simulink model "sim_quadrotor"  (R2015a)
settings: Solver=ode3  StartTime=0  StopTime=20  FixedStep=sampleTime_qcsim  MaxStep=0.1  RelTol=1e-3
InitFcn:
  | % load parameters of the default quadrotor
  | disp('Quadrotor parameters loaded by InitFcn')
  | paramsFilters %load mdl_quadcopter as well!
  | 
  | % change to Simulation folder if in data folder
  | cd([matlabpath '/Simulation']);
values from neighbouring files (symbols this model uses):
  altEstim =     [linsys1_pset3.mat]
  controlParams =     [linsys1_pset3.mat]
  ofhandle =     [linsys1_pset3.mat]
  quad =     [linsys1_pset3.mat]
  quadEDT =     [linsys1_pset3.mat]
  sampleTime_qcsim = 0.005    [linsys1_pset3.mat]
  vishandle =     [linsys1_pset3.mat]
undefined symbols (not defined in the file or in its folder): Discrete, K_poleplace, Time
libraries: simulink x26, ctrlSharedLib x3, commnoisgen2 x1
(part 2 of 2)

== system sim_quadrotor/DroneRS_Compensator/Estimator/EstimatorXYPosition/EstimatorXYPosition/OutlierHandling ==
  att_estimin : Inport
  posVIS_datin : Inport  Port=2
  pos_estim : Inport  Port=3
  Add1 : Sum  Inputs=+-
  Demux6 : Demux  Outputs=3
  Logical Operator3 : Logic  Inputs=4  AllPortsSameDT=off  OutDataTypeStr=boolean
  SelectX : Selector  InputPortWidth=4  Indices=[1]
  SelectXY : Selector  InputPortWidth=4  Indices=[1 2]
  abs : MATLAB Function  TreatAsAtomicUnit=on
  checkPosavailable : simulink/Logic and Bit Operations/Compare To Constant  relop=~=  const=-99  OutDataTypeStr=boolean
  maxp3 : simulink/Logic and Bit Operations/Compare To Constant  relop=<=  const=vishandle.att_UpperLimit  OutDataTypeStr=boolean
  maxq3 : simulink/Logic and Bit Operations/Compare To Constant  relop=<=  const=vishandle.att_UpperLimit  OutDataTypeStr=boolean
  planarjumpsVISPOS : simulink/Logic and Bit Operations/Compare To Constant  relop=<  const=vishandle.deltaXY  OutDataTypeStr=boolean
  enable_flag : Outport
  wires:
  att_estimin/1 -> Demux6/1
  posVIS_datin/1 -> SelectXY/1, SelectX/1
  SelectX/1 -> checkPosavailable/1
  checkPosavailable/1 -> Logical Operator3/1
  Logical Operator3/1 -> enable_flag/1
  Demux6/2 -> maxp3/1
  Demux6/3 -> maxq3/1
  maxp3/1 -> Logical Operator3/2
  maxq3/1 -> Logical Operator3/3
  SelectXY/1 -> Add1/1
  Add1/1 -> abs/1(vec)
  pos_estim/1 -> Add1/2
  abs/1(y) -> planarjumpsVISPOS/1
  planarjumpsVISPOS/1 -> Logical Operator3/4

== matlab function sim_quadrotor/Drone_Sensorsystem/camera/trafo_RTB2RSSensors_trans ==
  data: u input; y output
function y = fcn(u)
%inverse yaw-rotation
y = ([cos(pi/4) sin(pi/4) 0 ; -sin(pi/4) cos(pi/4) 0; 0 0 1]*u);

== matlab function sim_quadrotor/Drone_Sensorsystem/IMU_Pressure/trafo_RTB2RSSensors_trans ==
  data: u input; y output
function y = fcn(u)
%inverse yaw-rotation
y = ([cos(pi/4) sin(pi/4) 0 ; -sin(pi/4) cos(pi/4) 0; 0 0 1]*u);

== matlab function sim_quadrotor/Drone_Sensorsystem/IMU_Pressure/trafo_RTB2World_trans ==
  data: attitude input; vector input; y output
function y = fcn(attitude,vector)

yaw = attitude(1);
pitch = attitude(2);
roll = attitude(3);

R_RTBBody2Global =[ [ cos(pitch)*cos(yaw), cos(yaw)*sin(pitch)*sin(roll) - cos(roll)*sin(yaw), sin(roll)*sin(yaw) + cos(roll)*cos(yaw)*sin(pitch)];
[ cos(pitch)*sin(yaw), cos(roll)*cos(yaw) + sin(pitch)*sin(roll)*sin(yaw), cos(roll)*sin(pitch)*sin(yaw) - cos(yaw)*sin(roll)];
[         -sin(pitch),                               cos(pitch)*sin(roll),                               cos(pitch)*cos(roll)]];

% Rw_Global2RTBBody  = [0        sin(roll)          cos(roll);             %inverted Wronskian
%           0        cos(roll)*cos(pitch) -sin(roll)*cos(pitch);
%           cos(pitch) sin(roll)*sin(pitch) cos(roll)*sin(pitch)] / cos(pitch);
      
      
      
 y = R_RTBBody2Global*vector;      
      
%y = -([cos(pi/4) sin(pi/4); -sin(pi/4) cos(pi/4)]*u);

== matlab function sim_quadrotor/Drone_Sensorsystem/IMU_Pressure/trafo_World2RTB_trans1 ==
  data: attitude input; vector input; y output
function y = fcn(attitude,vector)

yaw = attitude(1);
pitch = attitude(2);
roll = attitude(3);

R_Global2RTBBody = [[                                cos(pitch)*cos(yaw),                                cos(pitch)*sin(yaw),          -sin(pitch)];
                    [ cos(yaw)*sin(pitch)*sin(roll) - cos(roll)*sin(yaw), cos(roll)*cos(yaw) + sin(pitch)*sin(roll)*sin(yaw), cos(pitch)*sin(roll)];
                    [ sin(roll)*sin(yaw) + cos(roll)*cos(yaw)*sin(pitch), cos(roll)*sin(pitch)*sin(yaw) - cos(yaw)*sin(roll), cos(pitch)*cos(roll)]];


% Rw_Global2RTBBody  = [0        sin(roll)          cos(roll);             %inverted Wronskian
%           0        cos(roll)*cos(pitch) -sin(roll)*cos(pitch);
%           cos(pitch) sin(roll)*sin(pitch) cos(roll)*sin(pitch)] / cos(pitch);
      
      
      
 y = R_Global2RTBBody*vector;      
      
%y = -([cos(pi/4) sin(pi/4); -sin(pi/4) cos(pi/4)]*u);

== matlab function sim_quadrotor/Drone_Sensorsystem/IMU_Pressure/trafo_RTB2RSSensors_rot1 ==
  data: u input; y output
function y = fcn(u)
%inverse yaw-rotation
y = [cos(pi/4)  sin(pi/4); -sin(pi/4) cos(pi/4)]*u;

== matlab function sim_quadrotor/DroneRS_Compensator/Estimator/EstimatorXYPosition/EstimatorVelocity/AccelerationWorld/World2Body ==
  data: attitude input; vector input; y output
function y = fcn(attitude,vector)

yaw = attitude(1);
pitch = attitude(2);
roll = attitude(3);

% rotz(yaw)*roty(pitch)*rotx(roll)
%     R_RTBBodytoGlobal = [cos(pitch)*cos(yaw) sin(roll)*sin(pitch)*cos(yaw)-cos(roll)*sin(yaw) cos(roll)*sin(pitch)*cos(yaw)+sin(roll)*sin(yaw);   %BBF > Inertial rotation matrix
%          cos(pitch)*sin(yaw) sin(roll)*sin(pitch)*sin(yaw)+cos(roll)*cos(yaw) cos(roll)*sin(pitch)*sin(yaw)-sin(roll)*cos(yaw);
%          -sin(pitch)         sin(roll)*cos(pitch)                            cos(roll)*cos(pitch)];
    

R_Global2RTBBody = [[                                cos(pitch)*cos(yaw),                                cos(pitch)*sin(yaw),          -sin(pitch)];
                    [ cos(yaw)*sin(pitch)*sin(roll) - cos(roll)*sin(yaw), cos(roll)*cos(yaw) + sin(pitch)*sin(roll)*sin(yaw), cos(pitch)*sin(roll)];
                    [ sin(roll)*sin(yaw) + cos(roll)*cos(yaw)*sin(pitch), cos(roll)*sin(pitch)*sin(yaw) - cos(yaw)*sin(roll), cos(pitch)*cos(roll)]];

% Rw_Global2RTBBody  = [0        sin(roll)          cos(roll);             %inverted Wronskian
%           0        cos(roll)*cos(pitch) -sin(roll)*cos(pitch);
%           cos(pitch) sin(roll)*sin(pitch) cos(roll)*sin(pitch)] / cos(pitch);
      
      
      
 y = R_Global2RTBBody*vector;      
      
%y = -([cos(pi/4) sin(pi/4); -sin(pi/4) cos(pi/4)]*u);

== matlab function sim_quadrotor/DroneRS_Compensator/Estimator/EstimatorXYPosition/EstimatorXYPosition/RStoWorld ==
  data: attitude input; vector input; vel_world output
function vel_world = fcn(attitude,vector)
yaw = attitude(1);
pitch = attitude(2);
roll = attitude(3);








R_RTBBodytoGlobal = [cos(pitch)*cos(yaw) sin(roll)*sin(pitch)*cos(yaw)-cos(roll)*sin(yaw) cos(roll)*sin(pitch)*cos(yaw)+sin(roll)*sin(yaw);   %BBF > Inertial rotation matrix
  cos(pitch)*sin(yaw) sin(roll)*sin(pitch)*sin(yaw)+cos(roll)*cos(yaw) cos(roll)*sin(pitch)*sin(yaw)-sin(roll)*cos(yaw);
  -sin(pitch)         sin(roll)*cos(pitch)                            cos(roll)*cos(pitch)];

vel_world = R_RTBBodytoGlobal*vector;

== matlab function sim_quadrotor/DroneRS_Compensator/Estimator/EstimatorAltitude/RStoWorldinacc ==
  data: attitude input; vector input; acc_world output
function acc_world = fcn(attitude,vector)
yaw = attitude(1);
pitch = attitude(2);
roll = attitude(3);








R_RTBBodytoGlobal = [cos(pitch)*cos(yaw) sin(roll)*sin(pitch)*cos(yaw)-cos(roll)*sin(yaw) cos(roll)*sin(pitch)*cos(yaw)+sin(roll)*sin(yaw);   %BBF > Inertial rotation matrix
  cos(pitch)*sin(yaw) sin(roll)*sin(pitch)*sin(yaw)+cos(roll)*cos(yaw) cos(roll)*sin(pitch)*sin(yaw)-sin(roll)*cos(yaw);
  -sin(pitch)         sin(roll)*cos(pitch)                            cos(roll)*cos(pitch)];

acc_world = R_RTBBodytoGlobal*vector;

== matlab function sim_quadrotor/DroneRS_Compensator/Estimator/EstimatorAltitude/WorldToRSinacc ==
  data: attitude input; vector input; acc_RS output
function acc_RS = fcn(attitude,vector)
yaw = attitude(1);
pitch = attitude(2);
roll = attitude(3);


R_Global2RTBBody = [[                                cos(pitch)*cos(yaw),                                cos(pitch)*sin(yaw),          -sin(pitch)];
                    [ cos(yaw)*sin(pitch)*sin(roll) - cos(roll)*sin(yaw), cos(roll)*cos(yaw) + sin(pitch)*sin(roll)*sin(yaw), cos(pitch)*sin(roll)];
                    [ sin(roll)*sin(yaw) + cos(roll)*cos(yaw)*sin(pitch), cos(roll)*sin(pitch)*sin(yaw) - cos(yaw)*sin(roll), cos(pitch)*cos(roll)]];

acc_RS = R_Global2RTBBody*vector;

== matlab function sim_quadrotor/DroneRS_Compensator/Estimator/EstimatorAttitude ==
  data: sensorIMU_datin input; yawVIS_datin input; validVIS_flagin input; gvecInit_datin input; att_estimout output; dt input; datt_estimout output; w_euler output
function [att_estimout,datt_estimout,w_euler] = fcn(sensorIMU_datin,yawVIS_datin,validVIS_flagin, gvecInit_datin,dt)
persistent yaw_cur pitch_cur roll_cur

p = sensorIMU_datin(4);
q = sensorIMU_datin(5);
r = sensorIMU_datin(6);

g = norm(gvecInit_datin,2);

if isempty(yaw_cur)
   yaw_cur = 0;
end
if isempty(pitch_cur)
   pitch_cur = 0;
end
if isempty(roll_cur)
   roll_cur = 0;
end


accvsGyro     = 0.001;
[yaw,pitch,roll,w_euler,forceMagnitudeApprox]= complimentaryfilter(yaw_cur, pitch_cur, roll_cur, g,dt,sensorIMU_datin, yawVIS_datin,validVIS_flagin,accvsGyro);
yaw_cur = yaw;
pitch_cur = pitch;
roll_cur = roll;

att_estimout = [yaw,pitch,roll]';
datt_estimout = [p,q,r]';

== matlab function sim_quadrotor/DroneRS_Compensator/Estimator/EstimatorXYPosition/EstimatorXYPosition/OutlierHandling/abs ==
  data: vec input; y output
function y = fcn(vec)
y = norm(vec,2);
